simulink model "Son_sim"  (R2022b)
settings: Solver=VariableStepAuto  StartTime=0.0  StopTime=90  RelTol=1e-3
undefined symbols (not defined in the file): Ad, Ag
libraries: audiosources x2, raspberrypiAVlib x1
settings Model: Creator=louxs  LastModifiedBy=mluser
settings OptimizationCC: DefaultParameterBehavior=Inlined  EnhancedBackFolding=on  PassReuseOutputArgsAs=Individual arguments  ZeroExternalMemoryAtStartup=off  ZeroInternalMemoryAtStartup=off  OptimizeBlockOrder=speed  DifferentSizesBufferReuse=on  OptimizationCustomize=off  EfficientTunableParamExpr=on
settings DebuggingCC: ParameterTunabilityLossMsg=error
settings ModelReferenceCC: EnableRefExpFcnMdlSchedulingChecks=on
settings SFSimCC: MATLABDynamicMemAlloc=off
settings RTWCC: Description=Embedded Coder  SystemTargetFile=ert.tlc  TemplateMakefile=ert_default_tmf
settings CodeAppCC: ForceParamTrailComments=on  IgnoreCustomStorageClasses=off  OperatorAnnotations=on  SimulinkDataObjDesc=on  SFDataObjDesc=on  InsertBlockDesc=on
settings ERTTargetCC: TargetLangStandard=C99 (ISO)  GenerateSampleERTMain=on  InlinedParameterPlacement=NonHierarchical  ERTCustomFileTemplate=example_file_process.tlc

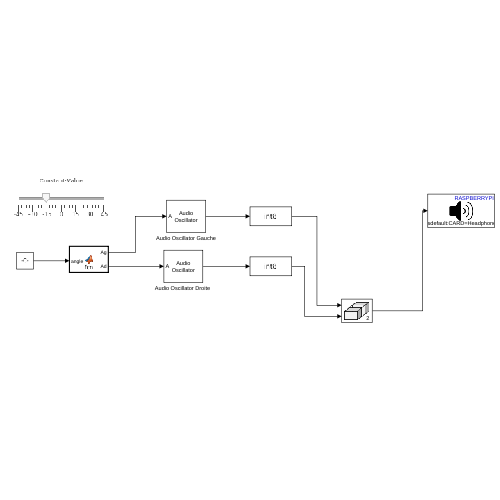
[thumbnail: Simulink's stored preview of the top-level diagram]
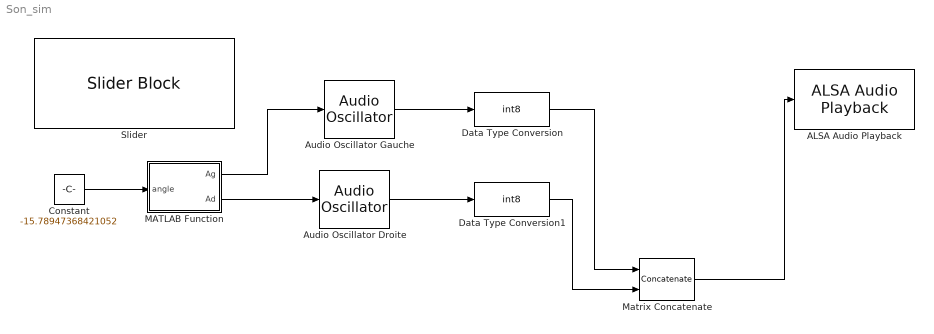
== system Son_sim ==
  ALSA Audio Playback : raspberrypiAVlib/ALSA Audio Playback  deviceStr=sysdefault:CARD=Headphones  sampleRateEnum=44100  queueDuration=0.5  blockPlatform=LINUX
  "Audio Oscillator Droite " : audiosources/Audio Oscillator  FrequencyPort=off  Frequency=350  AmplitudePort=on  Amplitude=Ag  DCOffsetPort=off  PhaseOffset=0  DCOffset=0  WidthPort=off  Width=1  DutyCyclePort=off  DutyCycle=0.5  SampsPerFrame=512  Fs=44100  OutputDataType=single  SimulateUsing=Code generation
      settings: SignalType=sine
  Audio Oscillator Gauche : audiosources/Audio Oscillator  FrequencyPort=off  Frequency=350  AmplitudePort=on  Amplitude=Ad  DCOffsetPort=off  PhaseOffset=0  DCOffset=0  WidthPort=off  Width=1  DutyCyclePort=off  DutyCycle=0.5  SampsPerFrame=512  Fs=44100  OutputDataType=double  SimulateUsing=Code generation
      settings: SignalType=sine
  Constant : Constant  Value=-15.78947368421052
  Data Type Conversion : DataTypeConversion  OutDataTypeStr=int8  SaturateOnIntegerOverflow=off  RndMeth=Floor
  Data Type Conversion1 : DataTypeConversion  OutDataTypeStr=int8  SaturateOnIntegerOverflow=off  RndMeth=Floor
  MATLAB Function : MATLAB Function  TreatAsAtomicUnit=on
  Matrix Concatenate : Concatenate  Mode=Multidimensional array  ConcatenateDimension=2
  Slider : SliderBlock  ScaleMin=-45  ScaleMax=45
  wires:
  Constant/1 -> MATLAB Function/1(angle)
  MATLAB Function/2(Ad) -> "Audio Oscillator Droite "/1
  MATLAB Function/1(Ag) -> Audio Oscillator Gauche/1
  Audio Oscillator Gauche/1 -> Data Type Conversion/1
  Data Type Conversion/1 -> Matrix Concatenate/1
  Matrix Concatenate/1 -> ALSA Audio Playback/1
  "Audio Oscillator Droite "/1 -> Data Type Conversion1/1
  Data Type Conversion1/1 -> Matrix Concatenate/2

== matlab function Son_sim/MATLAB Function ==
  data: Ag output; Ad output; angle input
function [Ag, Ad]= fcn(angle)
if angle > 0
    Ag = 0;
    Ad = 0.001*(angle^2);
else 
    Ag = 0.001*(angle^2);
    Ad = 0;
end
end
